simulink model "windup"  (R2019b)
settings: Solver=VariableStepAuto  StartTime=0.0  StopTime=80  RelTol=1e-3
values from neighbouring files (symbols this model uses):
  Ki = 0.2    [skrypt.m]
  Kp = 2    [skrypt.m]
  u_sat = 10    [skrypt.m]
  y_ref = 10    [skrypt.m]
settings Model: Creator=szymo  LastModifiedBy=szymo
settings SFSimCC: CustomCodeUndefinedFunction=UseInterfaceOnly

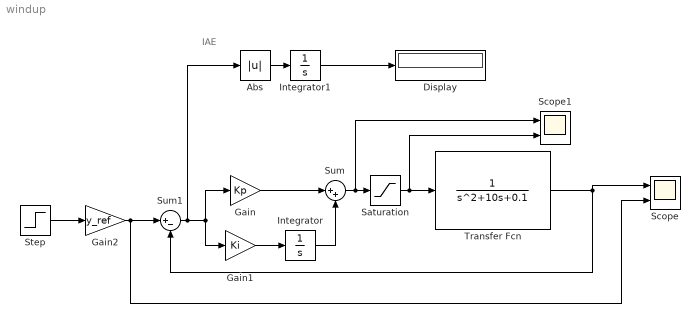
== system windup ==
  note: IAE
  Abs : Abs
  Display : Display
  Gain : Gain  Gain=Kp
  Gain1 : Gain  Gain=Ki
  Gain2 : Gain  Gain=y_ref
  Integrator : Integrator
  Integrator1 : Integrator
  Saturation : Saturate  UpperLimit=u_sat  LowerLimit=-u_sat
  Scope : Scope  NumInputPorts=2
  Scope1 : Scope  NumInputPorts=2
  Step : Step  SampleTime=0
  Sum : Sum  Inputs=|++
  Sum1 : Sum  Inputs=|+-
  Transfer Fcn : TransferFcn  Denominator=[1 10 0.1]
  wires:
  Gain1/1 -> Integrator/1
  Integrator/1 -> Sum/2
  Gain/1 -> Sum/1
  Sum/1 -> Scope1/1, Saturation/1
  Saturation/1 -> Scope1/2, Transfer Fcn/1
  Transfer Fcn/1 -> Sum1/2, Scope/1
  Sum1/1 -> Abs/1, Gain1/1, Gain/1
  Abs/1 -> Integrator1/1
  Integrator1/1 -> Display/1
  Step/1 -> Gain2/1
  Gain2/1 -> Scope/2, Sum1/1
